simulink model "Han_HQ_Sim_FB"  (Simulink 10.1)
settings: Solver=ode45  StartTime=0.0  StopTime=10  MaxStep=0.1  RelTol=1e-3  EnableMultiTasking=on
InitFcn:
  | AC=23; %Change to your assigned aircraft
  | SC_DynEqns;
  | X0=[U1 tht 0 tht 0 0 0 0]';
  | maneuver = 1;
  | Han_MK_CLAW;
StartFcn:
  | tic
StopFcn:
  | toctime=toc;
  | if maneuver <1.5
  | mkplot_Pitch
  | elseif maneuver <2.5
  | mkplot_Roll
  | else
  | mkplot_Yaw
  | end
undefined symbols (not defined in the file): A, Alt, B, d2r, fps2kt, K, K_pitch, K_roll, K_yaw, P1, P2, P3, pdoub, pdoub_t, r2d, rdoub, rdoub_t, tht, ydoub, ydoub_t, Z1, Z2, Z3
libraries: simulink x42
settings Model: Creator=bordignk  LastModifiedBy=Edward Han
settings DataIOCC: SignalLoggingSaveFormat=ModelDataLogs
settings OptimizationCC: ExpressionDepthLimit=2147483647  InitFltsAndDblsToZero=on
settings DebuggingCC: FcnCallInpInsideContextMsg=warning  UnconnectedInputMsg=none  UnconnectedOutputMsg=none  StateNameClashWarn=warning  SFExecutionAtInitializationDiag=warning
settings SFSimCC: SimParseCustomCode=off
settings ConfigComp: CovSFcnEnable=off

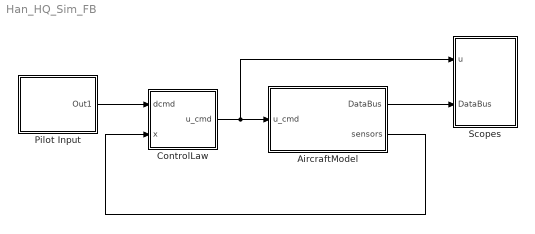
== system Han_HQ_Sim_FB ==
  AircraftModel : Subsystem
  ControlLaw : Subsystem
  Pilot Input : Subsystem
  Scopes : Subsystem
  wires:
  AircraftModel/1(DataBus) -> Scopes/2(DataBus)
  ControlLaw/1(u_cmd) -> AircraftModel/1(u_cmd), Scopes/1(u)
  AircraftModel/2(sensors) -> ControlLaw/2(x)
  Pilot Input/1(Out1) -> ControlLaw/1(dcmd)

== system Han_HQ_Sim_FB/AircraftModel ==
  u_cmd : Inport
  ControlLimits : Subsystem
  Gain : Gain  Gain=B  Multiplication=Matrix(K*u)
  Gain2 : Gain  Gain=A  Multiplication=Matrix(K*u)
  Integrator : Integrator  InitialCondition=zeros(8,1)
  Make_Data : Subsystem
  Sum : Sum  Inputs=|++
  DataBus : Outport
  sensors : Outport  Port=2
  wires:
  Gain2/1 -> Sum/2
  Sum/1 -> Integrator/1, Make_Data/1(xdt)  "xdt"
  Gain/1 -> Sum/1
  u_cmd/1 -> ControlLimits/1(u_cmd)
  Make_Data/1(DataBus) -> DataBus/1
  ControlLimits/1(u) -> Gain/1
  Integrator/1 -> Make_Data/2(x)  "x"
  Make_Data/2(x_out) -> sensors/1, Gain2/1

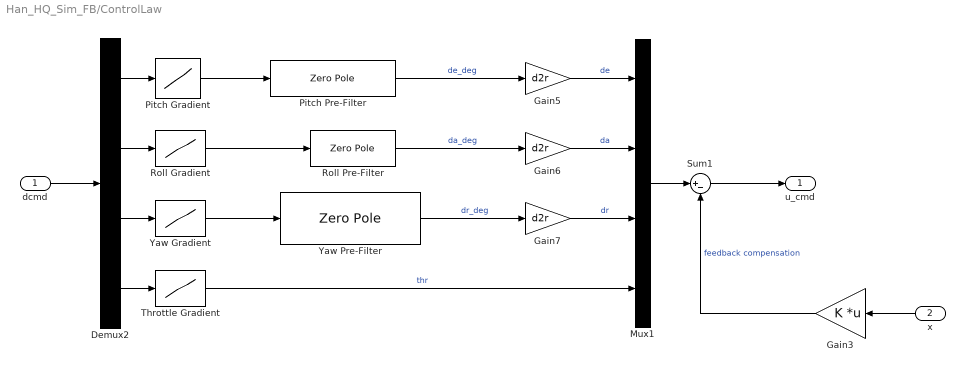
== system Han_HQ_Sim_FB/ControlLaw ==
  dcmd : Inport
  x : Inport  Port=2
  Demux2 : Demux
  Gain3 : Gain  Gain=K  Multiplication=Matrix(K*u)
  Gain5 : Gain  Gain=d2r
  Gain6 : Gain  Gain=d2r
  Gain7 : Gain  Gain=d2r
  Mux1 : Mux
  Pitch Gradient : Lookup  InputValues=[-1 1]  Table=[25 -25]  LookUpMeth=Interpolation-Use End Values
  Pitch Pre-Filter : ZeroPole  Zeros=[P1(3:4)]  Poles=Z1  Gain=K_pitch
  Roll Gradient : Lookup  InputValues=[-1 1]  Table=[-30 30]  LookUpMeth=Interpolation-Use End Values
  Roll Pre-Filter : ZeroPole  Zeros=[P2(4)]  Poles=Z2  Gain=K_roll
  Sum1 : Sum  Inputs=|+-
  Throttle Gradient : Lookup  InputValues=[-1 1]  Table=[5 -5]  LookUpMeth=Interpolation-Use End Values
  Yaw Gradient : Lookup  InputValues=[-1 1]  Table=[-30 30]  LookUpMeth=Interpolation-Use End Values
  Yaw Pre-Filter : ZeroPole  Zeros=[P3(4) P3(3)]  Poles=[Z3]  Gain=K_yaw
  u_cmd : Outport
  wires:
  Gain3/1 -> Sum1/2  "feedback compensation"
  Sum1/1 -> u_cmd/1
  x/1 -> Gain3/1
  Gain6/1 -> Mux1/2  "da"
  Gain7/1 -> Mux1/3  "dr"
  Demux2/2 -> Roll Gradient/1
  Demux2/4 -> Throttle Gradient/1
  Pitch Gradient/1 -> Pitch Pre-Filter/1
  Roll Gradient/1 -> Roll Pre-Filter/1
  Throttle Gradient/1 -> Mux1/4  "thr"
  Gain5/1 -> Mux1/1  "de"
  dcmd/1 -> Demux2/1
  Demux2/1 -> Pitch Gradient/1
  Mux1/1 -> Sum1/1
  Pitch Pre-Filter/1 -> Gain5/1  "de_deg"
  Roll Pre-Filter/1 -> Gain6/1  "da_deg"
  Yaw Gradient/1 -> Yaw Pre-Filter/1
  Demux2/3 -> Yaw Gradient/1
  Yaw Pre-Filter/1 -> Gain7/1  "dr_deg"

== system Han_HQ_Sim_FB/Pilot Input ==
  Mux : Mux
  Pitch Stick Sequence : Subsystem  mask{SEQ_t=pdoub_t, SEQ=pdoub}
      mask prompts: SEQ_t "Time values:"; SEQ "Output values:"
      mask Display: disp('Non-repeating\nSequence')
  Roll Stick Sequence : Subsystem  mask{SEQ_t=rdoub_t, SEQ=rdoub}
      mask prompts: SEQ_t "Time values:"; SEQ "Output values:"
      mask Display: disp('Non-repeating\nSequence')
  Rudder Pedal Sequence : Subsystem  mask{SEQ_t=ydoub_t, SEQ=ydoub}
      mask prompts: SEQ_t "Time values:"; SEQ "Output values:"
      mask Display: disp('Non-repeating\nSequence')
  Throttle Sequence : Subsystem  mask{SEQ_t=[0 25], SEQ=[0 0]}
      mask prompts: SEQ_t "Time values:"; SEQ "Output values:"
      mask Display: disp('Non-repeating\nSequence')
  To Workspace : ToWorkspace  VariableName=pilot_pitch  SampleTime=-1
  To Workspace1 : ToWorkspace  VariableName=pilot_roll  SampleTime=-1
  To Workspace2 : ToWorkspace  VariableName=pilot_rudder  SampleTime=-1
  To Workspace3 : ToWorkspace  VariableName=pilot_throttle  SampleTime=-1
  Out1 : Outport
  wires:
  Mux/1 -> Out1/1
  Pitch Stick Sequence/1(Out1) -> To Workspace/1, Mux/1  "dpitch"
  Rudder Pedal Sequence/1(Out1) -> Mux/3, To Workspace2/1  "dyaw"
  Roll Stick Sequence/1(Out1) -> To Workspace1/1, Mux/2  "droll"
  Throttle Sequence/1(Out1) -> Mux/4, To Workspace3/1  "dthr"

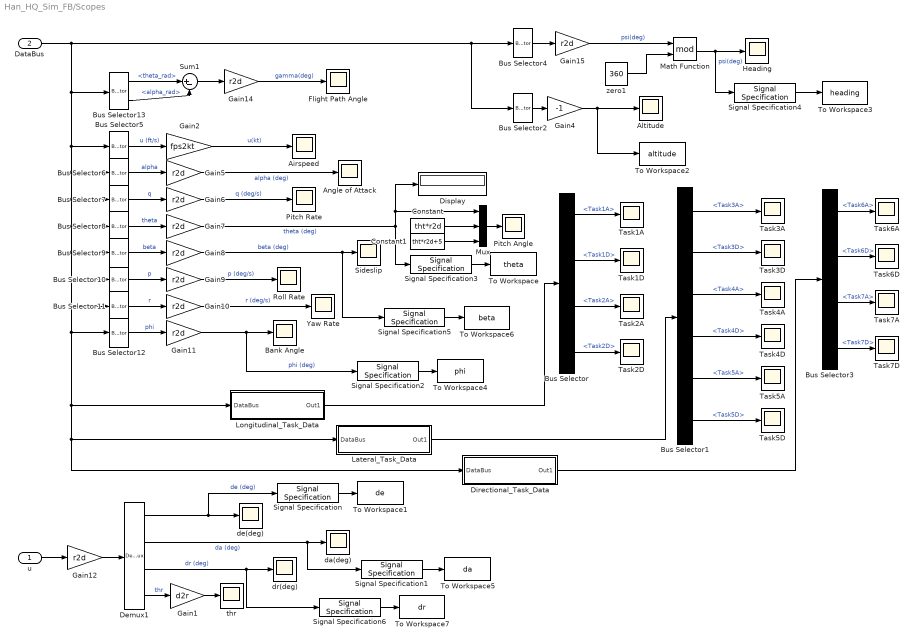
== system Han_HQ_Sim_FB/Scopes ==
  u : Inport
  DataBus : Inport  Port=2
  Airspeed : Scope
  Altitude : Scope
  Angle of Attack : Scope
  Bank Angle : Scope
  Bus Selector : BusSelector  OutputSignals=Task1A,Task1D,Task2A,Task2D
  Bus Selector1 : BusSelector  OutputSignals=Task3A,Task3D,Task4A,Task4D,Task5A,Task5D
  Bus Selector10 : BusSelector  OutputSignals=p_rps  OutputAsBus=on
  Bus Selector11 : BusSelector  OutputSignals=r_rps  OutputAsBus=on
  Bus Selector12 : BusSelector  OutputSignals=phi_rad  OutputAsBus=on
  Bus Selector13 : BusSelector  OutputSignals=theta_rad,alpha_rad
  Bus Selector2 : BusSelector  OutputSignals=ze_ft  OutputAsBus=on
  Bus Selector3 : BusSelector  OutputSignals=Task6A,Task6D,Task7A,Task7D
  Bus Selector4 : BusSelector  OutputSignals=psi_rad  OutputAsBus=on
  Bus Selector5 : BusSelector  OutputSignals=v_fps  OutputAsBus=on
  Bus Selector6 : BusSelector  OutputSignals=alpha_rad  OutputAsBus=on
  Bus Selector7 : BusSelector  OutputSignals=q_rps  OutputAsBus=on
  Bus Selector8 : BusSelector  OutputSignals=theta_rad  OutputAsBus=on
  Bus Selector9 : BusSelector  OutputSignals=beta_rad  OutputAsBus=on
  Constant : Constant  Value=tht*r2d
  Constant1 : Constant  Value=tht*r2d+5
  Demux1 : Demux
  Directional_Task_Data : Subsystem
  Display : Display
  Flight Path Angle : Scope
  Gain1 : Gain  Gain=d2r
  Gain{5..12,14..15} (10 alike) : Gain  Gain=r2d
  Gain2 : Gain  Gain=fps2kt
  Gain4 : Gain  Gain=-1
  Heading : Scope
  Lateral_Task_Data : Subsystem
  Longitudinal_Task_Data : Subsystem
  Math Function : Math  Operator=mod  SignedPower=on  SaturateOnIntegerOverflow=on
  Mux : Mux  Inputs=3
  Pitch Angle : Scope
  Pitch Rate : Scope
  Roll Rate : Scope
  Sideslip : Scope
  Signal Specification{,1..6} (7 alike) : SignalSpecification  Dimensions=[1]
  Sum1 : Sum  Inputs=|+-
  Task1A : Scope
  Task1D : Scope
  Task2A : Scope
  Task2D : Scope
  Task3A : Scope
  Task3D : Scope
  Task4A : Scope
  Task4D : Scope
  Task5A : Scope
  Task5D : Scope
  Task6A : Scope
  Task6D : Scope
  Task7A : Scope
  Task7D : Scope
  To Workspace : ToWorkspace  VariableName=theta  SampleTime=-1
  To Workspace1 : ToWorkspace  VariableName=de  SampleTime=-1
  To Workspace2 : ToWorkspace  VariableName=altitude  SampleTime=-1
  To Workspace3 : ToWorkspace  VariableName=heading  SampleTime=-1
  To Workspace4 : ToWorkspace  VariableName=phi  SampleTime=-1
  To Workspace5 : ToWorkspace  VariableName=da  SampleTime=-1
  To Workspace6 : ToWorkspace  VariableName=beta  SampleTime=-1
  To Workspace7 : ToWorkspace  VariableName=dr  SampleTime=-1
  Yaw Rate : Scope
  da(deg) : Scope
  de(deg) : Scope
  dr(deg) : Scope
  thr : Scope
  zero1 : Constant  Value=360
  wires:
  Gain12/1 -> Demux1/1
  Demux1/1 -> de(deg)/1, Signal Specification/1  "de (deg)"
  Demux1/2 -> da(deg)/1, Signal Specification1/1  "da (deg)"
  Demux1/3 -> dr(deg)/1, Signal Specification6/1  "dr (deg)"
  u/1 -> Gain12/1
  DataBus/1 -> Bus Selector5/1, Bus Selector6/1, Bus Selector7/1, Bus Selector8/1, Bus Selector9/1, Bus Selector10/1, Bus Selector11/1, Bus Selector12/1, Directional_Task_Data/1(DataBus), Lateral_Task_Data/1(DataBus), Longitudinal_Task_Data/1(DataBus), Bus Selector13/1, Bus Selector4/1, Bus Selector2/1
  Demux1/4 -> Gain1/1  "thr"
  Math Function/1 -> Heading/1, Signal Specification4/1  "psi(deg)"
  Bus Selector2/1 -> Gain4/1
  Gain4/1 -> Altitude/1, To Workspace2/1
  Bus Selector4/1 -> Gain15/1
  Bus Selector5/1 -> Gain2/1  "u (ft/s)"
  Bus Selector6/1 -> Gain5/1  "alpha"
  Bus Selector7/1 -> Gain6/1  "q"
  Bus Selector8/1 -> Gain7/1  "theta"
  Bus Selector9/1 -> Gain8/1  "beta"
  Bus Selector10/1 -> Gain9/1  "p"
  Bus Selector11/1 -> Gain10/1  "r"
  Bus Selector12/1 -> Gain11/1  "phi"
  Gain5/1 -> Angle of Attack/1  "alpha (deg)"
  Gain6/1 -> Pitch Rate/1  "q (deg/s)"
  Gain7/1 -> Signal Specification3/1, Display/1, Mux/1  "theta (deg)"
  Gain8/1 -> Sideslip/1, Signal Specification5/1  "beta (deg)"
  Gain9/1 -> Roll Rate/1  "p (deg/s)"
  Gain10/1 -> Yaw Rate/1  "r (deg/s)"
  Gain11/1 -> Bank Angle/1, Signal Specification2/1  "phi (deg)"
  Gain2/1 -> Airspeed/1  "u(kt)"
  Gain1/1 -> thr/1
  Gain15/1 -> Math Function/1  "psi(deg)"
  zero1/1 -> Math Function/2
  Gain14/1 -> Flight Path Angle/1  "gamma(deg)"
  Bus Selector13/1 -> Sum1/1  "<theta_rad>"
  Bus Selector13/2 -> Sum1/2  "<alpha_rad>"
  Sum1/1 -> Gain14/1
  Signal Specification/1 -> To Workspace1/1
  Signal Specification1/1 -> To Workspace5/1
  Signal Specification2/1 -> To Workspace4/1
  Signal Specification3/1 -> To Workspace/1
  Signal Specification4/1 -> To Workspace3/1
  Signal Specification5/1 -> To Workspace6/1
  Signal Specification6/1 -> To Workspace7/1
  Longitudinal_Task_Data/1(Out1) -> Bus Selector/1
  Bus Selector/1 -> Task1A/1  "<Task1A>"
  Bus Selector/2 -> Task1D/1  "<Task1D>"
  Bus Selector/3 -> Task2A/1  "<Task2A>"
  Bus Selector/4 -> Task2D/1  "<Task2D>"
  Lateral_Task_Data/1(Out1) -> Bus Selector1/1
  Bus Selector1/1 -> Task3A/1  "<Task3A>"
  Bus Selector1/2 -> Task3D/1  "<Task3D>"
  Bus Selector1/3 -> Task4A/1  "<Task4A>"
  Bus Selector1/4 -> Task4D/1  "<Task4D>"
  Bus Selector1/5 -> Task5A/1  "<Task5A>"
  Bus Selector1/6 -> Task5D/1  "<Task5D>"
  Directional_Task_Data/1(Out1) -> Bus Selector3/1
  Bus Selector3/1 -> Task6A/1  "<Task6A>"
  Bus Selector3/2 -> Task6D/1  "<Task6D>"
  Bus Selector3/3 -> Task7A/1  "<Task7A>"
  Bus Selector3/4 -> Task7D/1  "<Task7D>"
  Mux/1 -> Pitch Angle/1
  Constant/1 -> Mux/2
  Constant1/1 -> Mux/3

== system Han_HQ_Sim_FB/AircraftModel/ControlLimits ==
  u_cmd : Inport
  Demux2 : Demux
  Mux : Mux
  Saturation : Saturate  UpperLimit=25*d2r  LowerLimit=-25*d2r
  Saturation1 : Saturate  UpperLimit=30*d2r  LowerLimit=-30*d2r
  Saturation2 : Saturate  UpperLimit=30*d2r  LowerLimit=-30*d2r
  Saturation3 : Saturate  UpperLimit=5  LowerLimit=-5
  u : Outport
  wires:
  Demux2/1 -> Saturation/1
  Demux2/2 -> Saturation1/1
  Demux2/3 -> Saturation2/1
  Saturation/1 -> Mux/1
  Saturation1/1 -> Mux/2
  Saturation2/1 -> Mux/3
  Saturation3/1 -> Mux/4
  u_cmd/1 -> Demux2/1
  Mux/1 -> u/1
  Demux2/4 -> Saturation3/1

== system Han_HQ_Sim_FB/AircraftModel/Make_Data ==
  xdt : Inport  PortDimensions=[8 1]
  x : Inport  Port=2  PortDimensions=[8 1]
  Bus Selector : BusSelector  OutputSignals=v_fps,alpha_rad,q_rps,theta_rad,beta_rad,p_rps,r_rps,phi_rad  OutputAsBus=on
  Bus to Vector : BusToVector
  Constant : Constant  Value=X0
  Constant1 : Constant  Value=X0
  Earth Axis : Subsystem
  Subsystem2 : Subsystem
  Sum1 : Sum  Inputs=|++
  Sum2 : Sum  Inputs=|+-
  DataBus : Outport
  x_out : Outport  Port=2
  wires:
  x/1 -> Sum1/1
  Constant/1 -> Sum1/2
  Sum1/1 -> Subsystem2/1(x), Earth Axis/1(x)
  Earth Axis/2(xe) -> Subsystem2/3(Xe)
  xdt/1 -> Subsystem2/4(xdt)
  Subsystem2/1(DataBus) -> Bus Selector/1, DataBus/1
  Earth Axis/1(Ve) -> Subsystem2/2(Ve)
  Bus Selector/1 -> Bus to Vector/1
  Bus to Vector/1 -> Sum2/1
  Constant1/1 -> Sum2/2
  Sum2/1 -> x_out/1

== system Han_HQ_Sim_FB/Pilot Input/Pitch Stick Sequence ==
  Clock : Clock
  Lookup Table : Lookup  InputValues=SEQ_t  Table=SEQ  LookUpMeth=Interpolation-Use End Values
  Out1 : Outport
  wires:
  Clock/1 -> Lookup Table/1
  Lookup Table/1 -> Out1/1

== system Han_HQ_Sim_FB/Pilot Input/Roll Stick Sequence ==
  Clock : Clock
  Lookup Table : Lookup  InputValues=SEQ_t  Table=SEQ  LookUpMeth=Interpolation-Use End Values
  Out1 : Outport
  wires:
  Lookup Table/1 -> Out1/1
  Clock/1 -> Lookup Table/1

== system Han_HQ_Sim_FB/Pilot Input/Rudder Pedal Sequence ==
  Clock : Clock
  Lookup Table : Lookup  InputValues=SEQ_t  Table=SEQ  LookUpMeth=Interpolation-Use End Values
  Out1 : Outport
  wires:
  Clock/1 -> Lookup Table/1
  Lookup Table/1 -> Out1/1

== system Han_HQ_Sim_FB/Pilot Input/Throttle Sequence ==
  Clock : Clock
  Lookup Table : Lookup  InputValues=SEQ_t  Table=SEQ  LookUpMeth=Interpolation-Use End Values
  Out1 : Outport
  wires:
  Lookup Table/1 -> Out1/1
  Clock/1 -> Lookup Table/1

== system Han_HQ_Sim_FB/Scopes/Directional_Task_Data ==
  DataBus : Inport
  Bus Creator : BusCreator  Inputs=4
  Bus Selector1 : BusSelector  OutputSignals=beta_rad
  Gain2 : Gain  Gain=r2d
  Task6 : Subsystem
  Task7 : Subsystem
  Out1 : Outport
  wires:
  Gain2/1 -> Task6/1(In1), Task7/2(In2)  "beta_deg"
  Bus Selector1/1 -> Gain2/1  "<beta_rad>"
  DataBus/1 -> Bus Selector1/1
  Bus Creator/1 -> Out1/1
  Task6/1(Task6D) -> Bus Creator/1
  Task6/2(Task6A) -> Task7/1(In1), Bus Creator/2
  Task7/1(Task7D) -> Bus Creator/3
  Task7/2(Task7A) -> Bus Creator/4

== system Han_HQ_Sim_FB/Scopes/Lateral_Task_Data ==
  DataBus : Inport
  Bus Creator : BusCreator  Inputs=6
  Bus Selector1 : BusSelector  OutputSignals=phi_rad
  Gain2 : Gain  Gain=r2d
  Task3 : Subsystem
  Task4 : Subsystem
  Task5 : Subsystem
  Out1 : Outport
  wires:
  DataBus/1 -> Bus Selector1/1
  Bus Selector1/1 -> Gain2/1  "<phi_rad>"
  Gain2/1 -> Task3/1(In1), Task4/2(In2), Task5/2(In2)  "phi_deg"
  Task3/2(Task3A) -> Task4/1(In1), Bus Creator/2
  Bus Creator/1 -> Out1/1
  Task3/1(Task3D) -> Bus Creator/1
  Task4/1(Task4D) -> Bus Creator/3
  Task5/1(Task5A) -> Bus Creator/5
  Task5/2(Task5D) -> Bus Creator/6
  Task4/2(Task4A) -> Task5/1(In1), Bus Creator/4

== system Han_HQ_Sim_FB/Scopes/Longitudinal_Task_Data ==
  DataBus : Inport
  Bus Creator : BusCreator  Inputs=4
  Bus Selector1 : BusSelector  OutputSignals=theta_rad  OutputAsBus=on
  Gain6 : Gain  Gain=r2d
  Task1 : Subsystem
  Task2 : Subsystem
  Out1 : Outport
  wires:
  DataBus/1 -> Bus Selector1/1
  Bus Selector1/1 -> Gain6/1
  Gain6/1 -> Task1/1(In1), Task2/2(In1)
  Task1/2(Task1A) -> Task2/1(In2), Bus Creator/2
  Task2/1(Task2A) -> Bus Creator/3
  Task2/2(Task2D) -> Bus Creator/4
  Bus Creator/1 -> Out1/1
  Task1/1(Task1D) -> Bus Creator/1

== system Han_HQ_Sim_FB/AircraftModel/Make_Data/Earth Axis ==
  x : Inport
  Selector : Selector  InputPortWidth=8  IndexOptions=Index vector (dialog)  Indices=[6 3 7]  OutputSizes=1
  Subsystem : Subsystem
  Subsystem1 : Subsystem
  Transpose : Math  Operator=transpose  SignedPower=on  SaturateOnIntegerOverflow=on
  uvw_body : Subsystem
  xe,ye,ze : Integrator  InitialCondition=[0 0 -Alt]
  Ve : Outport
  xe : Outport  Port=2
  wires:
  Subsystem1/1(DCM) -> Transpose/1
  Transpose/1 -> Subsystem/2(transform coefficients)
  Selector/1 -> Subsystem1/1("p q r ")
  uvw_body/1(Out1) -> Subsystem/1(x y z)
  x/1 -> Selector/1, uvw_body/1(In1)
  xe,ye,ze/1 -> xe/1
  Subsystem/1(Ve1) -> Ve/1, xe,ye,ze/1

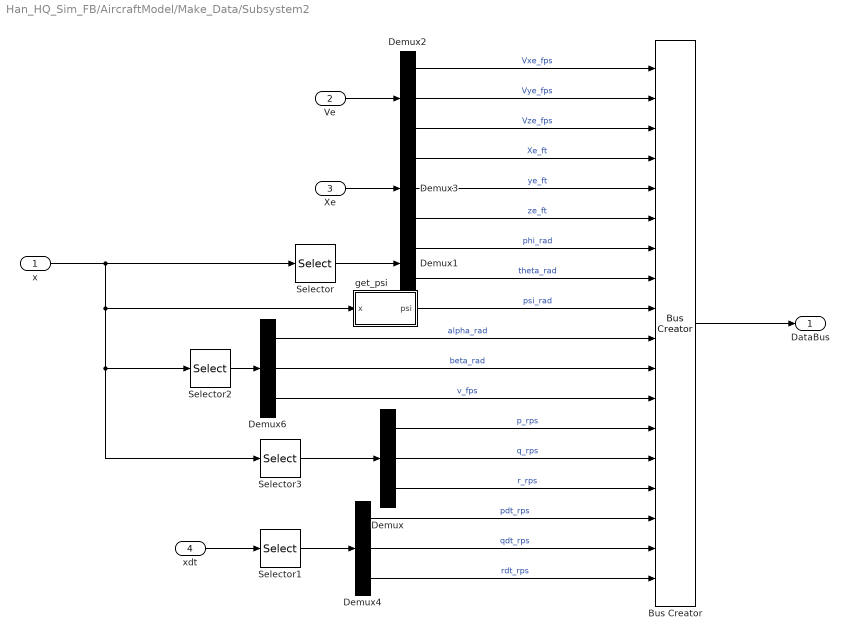
== system Han_HQ_Sim_FB/AircraftModel/Make_Data/Subsystem2 ==
  x : Inport
  Ve : Inport  Port=2
  Xe : Inport  Port=3
  xdt : Inport  Port=4
  Bus Creator : BusCreator  Inputs=18
  Demux{,2..4,6} (5 alike) : Demux  Outputs=3
  Demux1 : Demux  Outputs=2
  Selector : Selector  InputPortWidth=8  IndexOptions=Index vector (dialog)  Indices=[8 4]  OutputSizes=1
  Selector1 : Selector  InputPortWidth=8  IndexOptions=Index vector (dialog)  Indices=[6 3 7]  OutputSizes=1
  Selector2 : Selector  InputPortWidth=8  IndexOptions=Index vector (dialog)  Indices=[2 5 1]  OutputSizes=1
  Selector3 : Selector  InputPortWidth=8  IndexOptions=Index vector (dialog)  Indices=[6 3 7]  OutputSizes=1
  get_psi : Subsystem
  DataBus : Outport
  wires:
  Selector2/1 -> Demux6/1
  Selector/1 -> Demux1/1
  x/1 -> get_psi/1(x), Selector3/1, Selector2/1, Selector/1
  Demux4/3 -> Bus Creator/18  "rdt_rps"
  Demux4/2 -> Bus Creator/17  "qdt_rps"
  Demux4/1 -> Bus Creator/16  "pdt_rps"
  Demux/3 -> Bus Creator/15  "r_rps"
  Demux/2 -> Bus Creator/14  "q_rps"
  Demux/1 -> Bus Creator/13  "p_rps"
  Demux6/3 -> Bus Creator/12  "v_fps"
  Demux6/2 -> Bus Creator/11  "beta_rad"
  Demux6/1 -> Bus Creator/10  "alpha_rad"
  get_psi/1(psi) -> Bus Creator/9  "psi_rad"
  Demux1/2 -> Bus Creator/8  "theta_rad"
  Demux1/1 -> Bus Creator/7  "phi_rad"
  Demux3/3 -> Bus Creator/6  "ze_ft"
  Demux3/2 -> Bus Creator/5  "ye_ft"
  Demux3/1 -> Bus Creator/4  "Xe_ft"
  Demux2/3 -> Bus Creator/3  "Vze_fps"
  Demux2/2 -> Bus Creator/2  "Vye_fps"
  Demux2/1 -> Bus Creator/1  "Vxe_fps"
  xdt/1 -> Selector1/1
  Xe/1 -> Demux3/1
  Ve/1 -> Demux2/1
  Bus Creator/1 -> DataBus/1
  Selector3/1 -> Demux/1
  Selector1/1 -> Demux4/1

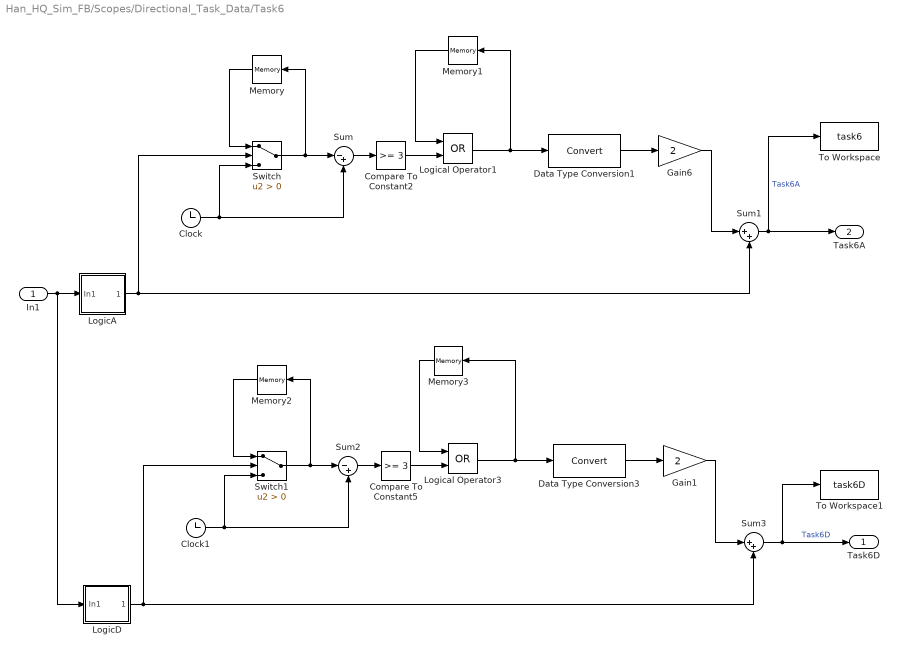
== system Han_HQ_Sim_FB/Scopes/Directional_Task_Data/Task6 ==
  In1 : Inport
  Clock : Clock
  Clock1 : Clock
  Compare To Constant2 : simulink/Logic and Bit Operations/Compare To Constant  relop=>=  const=3  OutDataTypeStr=uint8  ZeroCross=off
  Compare To Constant5 : simulink/Logic and Bit Operations/Compare To Constant  relop=>=  const=3  OutDataTypeStr=uint8  ZeroCross=off
  Data Type Conversion1 : DataTypeConversion
  Data Type Conversion3 : DataTypeConversion
  Gain1 : Gain  Gain=2
  Gain6 : Gain  Gain=2
  LogicA : Subsystem
  LogicD : Subsystem
  Logical Operator1 : Logic  Operator=OR  AllPortsSameDT=off  OutDataTypeStr=boolean
  Logical Operator3 : Logic  Operator=OR  AllPortsSameDT=off  OutDataTypeStr=boolean
  Memory{,1..3} (4 alike) : Memory
  Sum : Sum  Inputs=|-+
  Sum1 : Sum  Inputs=|++
  Sum2 : Sum  Inputs=|-+
  Sum3 : Sum  Inputs=|++
  Switch : Switch  Criteria=u2 > Threshold
  Switch1 : Switch  Criteria=u2 > Threshold
  To Workspace : ToWorkspace  VariableName=task6  SampleTime=-1
  To Workspace1 : ToWorkspace  VariableName=task6D  SampleTime=-1
  Task6D : Outport
  Task6A : Outport  Port=2
  wires:
  LogicD/1(Out1) -> Switch1/2, Sum3/2
  Gain1/1 -> Sum3/1
  Data Type Conversion3/1 -> Gain1/1
  Sum3/1 -> To Workspace1/1, Task6D/1  "Task6D"
  Memory3/1 -> Logical Operator3/1
  Logical Operator3/1 -> Memory3/1, Data Type Conversion3/1
  Compare To Constant5/1 -> Logical Operator3/2
  Sum2/1 -> Compare To Constant5/1
  Memory2/1 -> Switch1/1
  Switch1/1 -> Sum2/1, Memory2/1
  Clock1/1 -> Sum2/2, Switch1/3
  LogicA/1(Out1) -> Switch/2, Sum1/2
  Gain6/1 -> Sum1/1
  Data Type Conversion1/1 -> Gain6/1
  Sum1/1 -> Task6A/1, To Workspace/1  "Task6A"
  Memory1/1 -> Logical Operator1/1
  Logical Operator1/1 -> Memory1/1, Data Type Conversion1/1
  Compare To Constant2/1 -> Logical Operator1/2
  Sum/1 -> Compare To Constant2/1
  Memory/1 -> Switch/1
  Switch/1 -> Sum/1, Memory/1
  Clock/1 -> Sum/2, Switch/3
  In1/1 -> LogicD/1(In1), LogicA/1(In1)

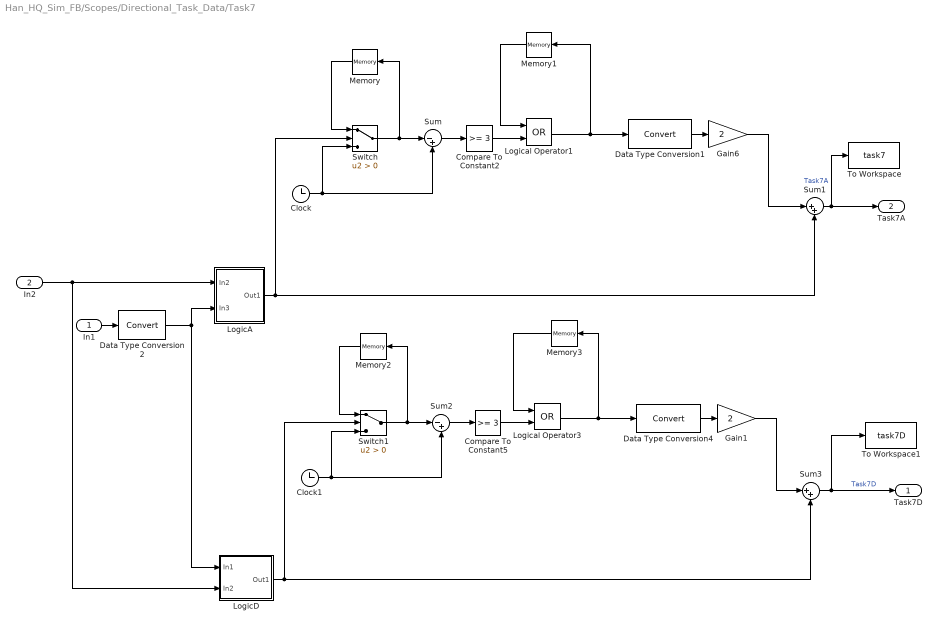
== system Han_HQ_Sim_FB/Scopes/Directional_Task_Data/Task7 ==
  In1 : Inport
  In2 : Inport  Port=2
  Clock : Clock
  Clock1 : Clock
  Compare To Constant2 : simulink/Logic and Bit Operations/Compare To Constant  relop=>=  const=3  OutDataTypeStr=uint8  ZeroCross=off
  Compare To Constant5 : simulink/Logic and Bit Operations/Compare To Constant  relop=>=  const=3  OutDataTypeStr=uint8  ZeroCross=off
  Data Type Conversion1 : DataTypeConversion
  Data Type Conversion2 : DataTypeConversion
  Data Type Conversion4 : DataTypeConversion
  Gain1 : Gain  Gain=2
  Gain6 : Gain  Gain=2
  LogicA : Subsystem
  LogicD : Subsystem
  Logical Operator1 : Logic  Operator=OR  AllPortsSameDT=off  OutDataTypeStr=boolean
  Logical Operator3 : Logic  Operator=OR  AllPortsSameDT=off  OutDataTypeStr=boolean
  Memory{,1..3} (4 alike) : Memory
  Sum : Sum  Inputs=|-+
  Sum1 : Sum  Inputs=|++
  Sum2 : Sum  Inputs=|-+
  Sum3 : Sum  Inputs=|++
  Switch : Switch  Criteria=u2 > Threshold
  Switch1 : Switch  Criteria=u2 > Threshold
  To Workspace : ToWorkspace  VariableName=task7  SampleTime=-1
  To Workspace1 : ToWorkspace  VariableName=task7D  SampleTime=-1
  Task7D : Outport
  Task7A : Outport  Port=2
  wires:
  Gain1/1 -> Sum3/1
  Data Type Conversion4/1 -> Gain1/1
  Sum3/1 -> To Workspace1/1, Task7D/1  "Task7D"
  Memory3/1 -> Logical Operator3/1
  Logical Operator3/1 -> Memory3/1, Data Type Conversion4/1
  Compare To Constant5/1 -> Logical Operator3/2
  Sum2/1 -> Compare To Constant5/1
  Memory2/1 -> Switch1/1
  Switch1/1 -> Sum2/1, Memory2/1
  Clock1/1 -> Sum2/2, Switch1/3
  LogicD/1(Out1) -> Sum3/2, Switch1/2
  Data Type Conversion2/1 -> LogicA/2(In3), LogicD/1(In1)
  Gain6/1 -> Sum1/1
  Data Type Conversion1/1 -> Gain6/1
  In1/1 -> Data Type Conversion2/1
  Sum1/1 -> To Workspace/1, Task7A/1  "Task7A"
  Memory1/1 -> Logical Operator1/1
  Logical Operator1/1 -> Memory1/1, Data Type Conversion1/1
  Compare To Constant2/1 -> Logical Operator1/2
  Sum/1 -> Compare To Constant2/1
  Memory/1 -> Switch/1
  Switch/1 -> Sum/1, Memory/1
  Clock/1 -> Sum/2, Switch/3
  In2/1 -> LogicD/2(In2), LogicA/1(In2)
  LogicA/1(Out1) -> Sum1/2, Switch/2

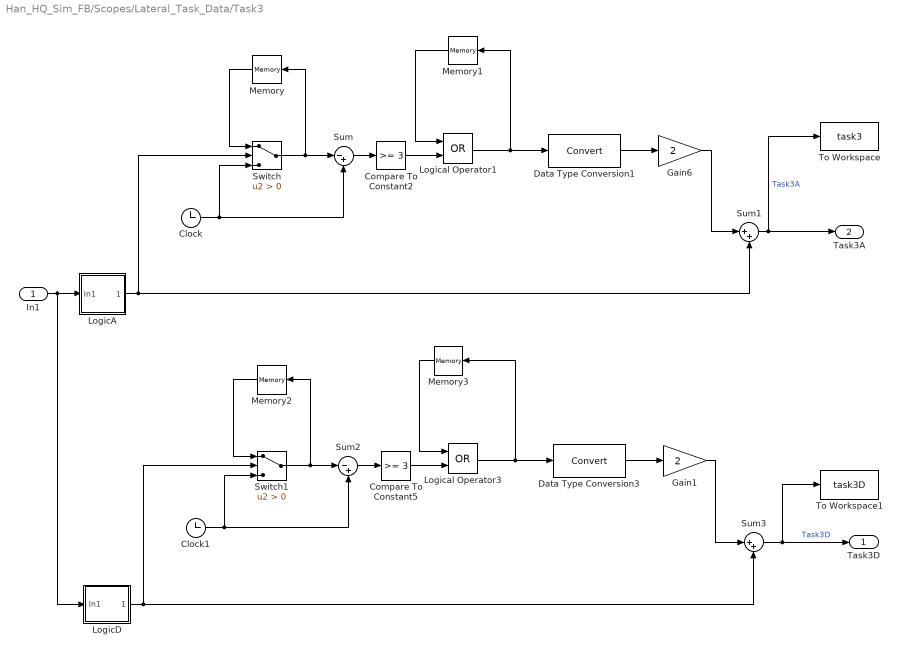
== system Han_HQ_Sim_FB/Scopes/Lateral_Task_Data/Task3 ==
  In1 : Inport
  Clock : Clock
  Clock1 : Clock
  Compare To Constant2 : simulink/Logic and Bit Operations/Compare To Constant  relop=>=  const=3  OutDataTypeStr=uint8  ZeroCross=off
  Compare To Constant5 : simulink/Logic and Bit Operations/Compare To Constant  relop=>=  const=3  OutDataTypeStr=uint8  ZeroCross=off
  Data Type Conversion1 : DataTypeConversion
  Data Type Conversion3 : DataTypeConversion
  Gain1 : Gain  Gain=2
  Gain6 : Gain  Gain=2
  LogicA : Subsystem
  LogicD : Subsystem
  Logical Operator1 : Logic  Operator=OR  AllPortsSameDT=off  OutDataTypeStr=boolean
  Logical Operator3 : Logic  Operator=OR  AllPortsSameDT=off  OutDataTypeStr=boolean
  Memory{,1..3} (4 alike) : Memory
  Sum : Sum  Inputs=|-+
  Sum1 : Sum  Inputs=|++
  Sum2 : Sum  Inputs=|-+
  Sum3 : Sum  Inputs=|++
  Switch : Switch  Criteria=u2 > Threshold
  Switch1 : Switch  Criteria=u2 > Threshold
  To Workspace : ToWorkspace  VariableName=task3  SampleTime=-1
  To Workspace1 : ToWorkspace  VariableName=task3D  SampleTime=-1
  Task3D : Outport
  Task3A : Outport  Port=2
  wires:
  In1/1 -> LogicA/1(In1), LogicD/1(In1)
  Clock/1 -> Switch/3, Sum/2
  Switch/1 -> Memory/1, Sum/1
  Memory/1 -> Switch/1
  Sum/1 -> Compare To Constant2/1
  Compare To Constant2/1 -> Logical Operator1/2
  Logical Operator1/1 -> Data Type Conversion1/1, Memory1/1
  Memory1/1 -> Logical Operator1/1
  Sum1/1 -> Task3A/1, To Workspace/1  "Task3A"
  Data Type Conversion1/1 -> Gain6/1
  Gain6/1 -> Sum1/1
  LogicA/1(Out1) -> Sum1/2, Switch/2
  Clock1/1 -> Switch1/3, Sum2/2
  Switch1/1 -> Memory2/1, Sum2/1
  Memory2/1 -> Switch1/1
  Sum2/1 -> Compare To Constant5/1
  Compare To Constant5/1 -> Logical Operator3/2
  Logical Operator3/1 -> Data Type Conversion3/1, Memory3/1
  Memory3/1 -> Logical Operator3/1
  Sum3/1 -> To Workspace1/1, Task3D/1  "Task3D"
  Data Type Conversion3/1 -> Gain1/1
  Gain1/1 -> Sum3/1
  LogicD/1(Out1) -> Sum3/2, Switch1/2

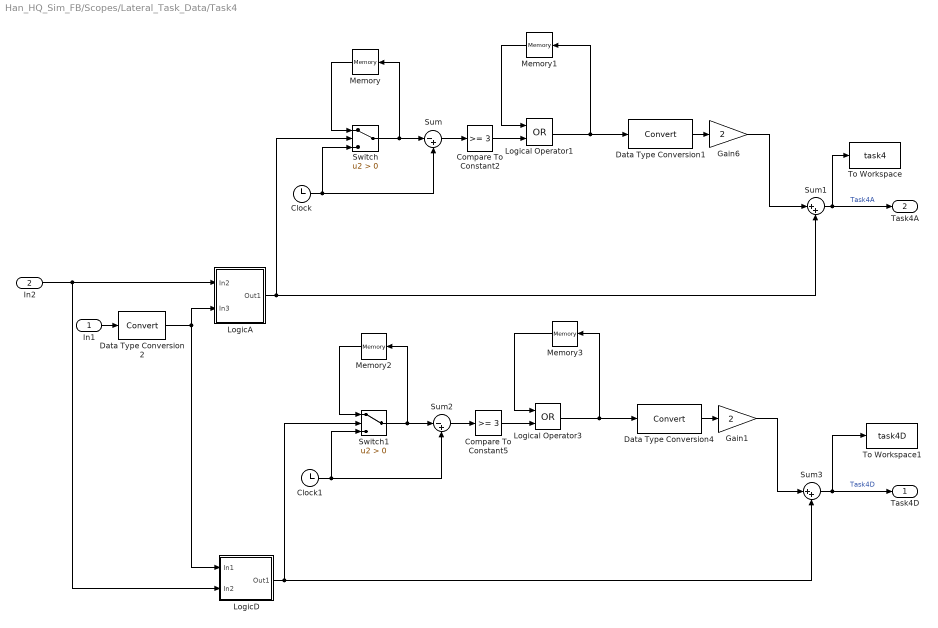
== system Han_HQ_Sim_FB/Scopes/Lateral_Task_Data/Task4 ==
  In1 : Inport
  In2 : Inport  Port=2
  Clock : Clock
  Clock1 : Clock
  Compare To Constant2 : simulink/Logic and Bit Operations/Compare To Constant  relop=>=  const=3  OutDataTypeStr=uint8  ZeroCross=off
  Compare To Constant5 : simulink/Logic and Bit Operations/Compare To Constant  relop=>=  const=3  OutDataTypeStr=uint8  ZeroCross=off
  Data Type Conversion1 : DataTypeConversion
  Data Type Conversion2 : DataTypeConversion
  Data Type Conversion4 : DataTypeConversion
  Gain1 : Gain  Gain=2
  Gain6 : Gain  Gain=2
  LogicA : Subsystem
  LogicD : Subsystem
  Logical Operator1 : Logic  Operator=OR  AllPortsSameDT=off  OutDataTypeStr=boolean
  Logical Operator3 : Logic  Operator=OR  AllPortsSameDT=off  OutDataTypeStr=boolean
  Memory{,1..3} (4 alike) : Memory
  Sum : Sum  Inputs=|-+
  Sum1 : Sum  Inputs=|++
  Sum2 : Sum  Inputs=|-+
  Sum3 : Sum  Inputs=|++
  Switch : Switch  Criteria=u2 > Threshold
  Switch1 : Switch  Criteria=u2 > Threshold
  To Workspace : ToWorkspace  VariableName=task4  SampleTime=-1
  To Workspace1 : ToWorkspace  VariableName=task4D  SampleTime=-1
  Task4D : Outport
  Task4A : Outport  Port=2
  wires:
  LogicA/1(Out1) -> Switch/2, Sum1/2
  In2/1 -> LogicA/1(In2), LogicD/2(In2)
  Clock/1 -> Switch/3, Sum/2
  Switch/1 -> Memory/1, Sum/1
  Memory/1 -> Switch/1
  Sum/1 -> Compare To Constant2/1
  Compare To Constant2/1 -> Logical Operator1/2
  Logical Operator1/1 -> Data Type Conversion1/1, Memory1/1
  Memory1/1 -> Logical Operator1/1
  Sum1/1 -> To Workspace/1, Task4A/1  "Task4A"
  In1/1 -> Data Type Conversion2/1
  Data Type Conversion1/1 -> Gain6/1
  Gain6/1 -> Sum1/1
  Data Type Conversion2/1 -> LogicD/1(In1), LogicA/2(In3)
  LogicD/1(Out1) -> Switch1/2, Sum3/2
  Clock1/1 -> Switch1/3, Sum2/2
  Switch1/1 -> Memory2/1, Sum2/1
  Memory2/1 -> Switch1/1
  Sum2/1 -> Compare To Constant5/1
  Compare To Constant5/1 -> Logical Operator3/2
  Logical Operator3/1 -> Data Type Conversion4/1, Memory3/1
  Memory3/1 -> Logical Operator3/1
  Sum3/1 -> To Workspace1/1, Task4D/1  "Task4D"
  Data Type Conversion4/1 -> Gain1/1
  Gain1/1 -> Sum3/1

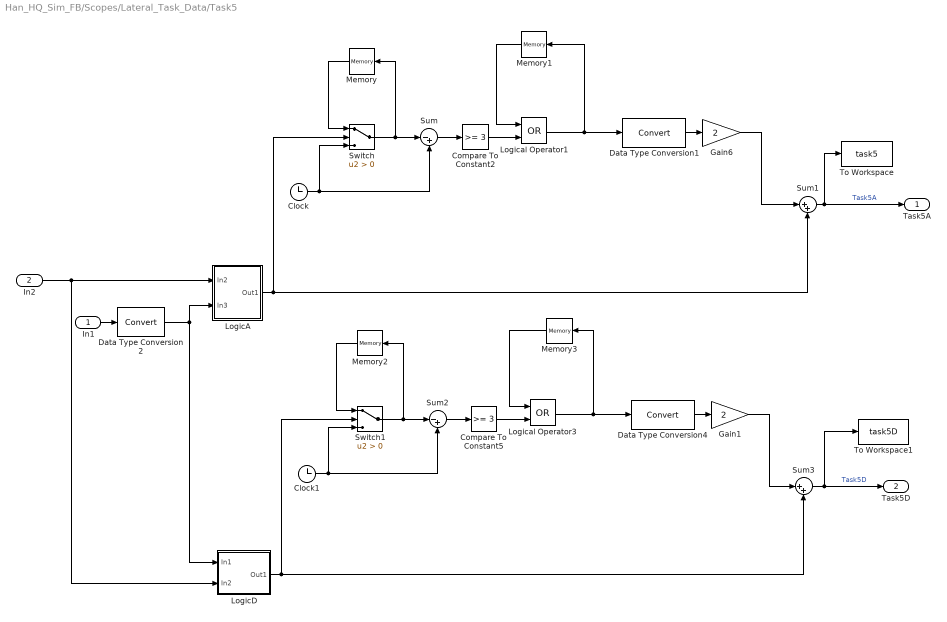
== system Han_HQ_Sim_FB/Scopes/Lateral_Task_Data/Task5 ==
  In1 : Inport
  In2 : Inport  Port=2
  Clock : Clock
  Clock1 : Clock
  Compare To Constant2 : simulink/Logic and Bit Operations/Compare To Constant  relop=>=  const=3  OutDataTypeStr=uint8  ZeroCross=off
  Compare To Constant5 : simulink/Logic and Bit Operations/Compare To Constant  relop=>=  const=3  OutDataTypeStr=uint8  ZeroCross=off
  Data Type Conversion1 : DataTypeConversion
  Data Type Conversion2 : DataTypeConversion
  Data Type Conversion4 : DataTypeConversion
  Gain1 : Gain  Gain=2
  Gain6 : Gain  Gain=2
  LogicA : Subsystem
  LogicD : Subsystem
  Logical Operator1 : Logic  Operator=OR  AllPortsSameDT=off  OutDataTypeStr=boolean
  Logical Operator3 : Logic  Operator=OR  AllPortsSameDT=off  OutDataTypeStr=boolean
  Memory{,1..3} (4 alike) : Memory
  Sum : Sum  Inputs=|-+
  Sum1 : Sum  Inputs=|++
  Sum2 : Sum  Inputs=|-+
  Sum3 : Sum  Inputs=|++
  Switch : Switch  Criteria=u2 > Threshold
  Switch1 : Switch  Criteria=u2 > Threshold
  To Workspace : ToWorkspace  VariableName=task5  SampleTime=-1
  To Workspace1 : ToWorkspace  VariableName=task5D  SampleTime=-1
  Task5A : Outport
  Task5D : Outport  Port=2
  wires:
  LogicA/1(Out1) -> Switch/2, Sum1/2
  In2/1 -> LogicA/1(In2), LogicD/2(In2)
  Clock/1 -> Switch/3, Sum/2
  Switch/1 -> Memory/1, Sum/1
  Memory/1 -> Switch/1
  Sum/1 -> Compare To Constant2/1
  Compare To Constant2/1 -> Logical Operator1/2
  Logical Operator1/1 -> Data Type Conversion1/1, Memory1/1
  Memory1/1 -> Logical Operator1/1
  Sum1/1 -> To Workspace/1, Task5A/1  "Task5A"
  In1/1 -> Data Type Conversion2/1
  Data Type Conversion1/1 -> Gain6/1
  Gain6/1 -> Sum1/1
  Data Type Conversion2/1 -> LogicD/1(In1), LogicA/2(In3)
  LogicD/1(Out1) -> Switch1/2, Sum3/2
  Clock1/1 -> Switch1/3, Sum2/2
  Switch1/1 -> Memory2/1, Sum2/1
  Memory2/1 -> Switch1/1
  Sum2/1 -> Compare To Constant5/1
  Compare To Constant5/1 -> Logical Operator3/2
  Logical Operator3/1 -> Data Type Conversion4/1, Memory3/1
  Memory3/1 -> Logical Operator3/1
  Sum3/1 -> To Workspace1/1, Task5D/1  "Task5D"
  Data Type Conversion4/1 -> Gain1/1
  Gain1/1 -> Sum3/1

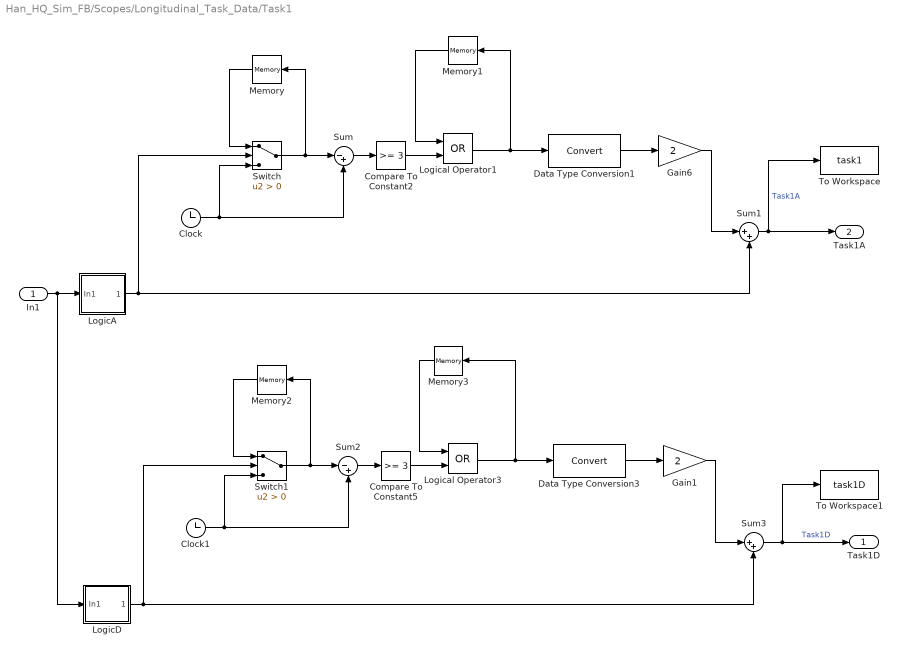
== system Han_HQ_Sim_FB/Scopes/Longitudinal_Task_Data/Task1 ==
  In1 : Inport
  Clock : Clock
  Clock1 : Clock
  Compare To Constant2 : simulink/Logic and Bit Operations/Compare To Constant  relop=>=  const=3  OutDataTypeStr=uint8  ZeroCross=off
  Compare To Constant5 : simulink/Logic and Bit Operations/Compare To Constant  relop=>=  const=3  OutDataTypeStr=uint8  ZeroCross=off
  Data Type Conversion1 : DataTypeConversion
  Data Type Conversion3 : DataTypeConversion
  Gain1 : Gain  Gain=2
  Gain6 : Gain  Gain=2
  LogicA : Subsystem
  LogicD : Subsystem
  Logical Operator1 : Logic  Operator=OR  AllPortsSameDT=off  OutDataTypeStr=boolean
  Logical Operator3 : Logic  Operator=OR  AllPortsSameDT=off  OutDataTypeStr=boolean
  Memory{,1..3} (4 alike) : Memory
  Sum : Sum  Inputs=|-+
  Sum1 : Sum  Inputs=|++
  Sum2 : Sum  Inputs=|-+
  Sum3 : Sum  Inputs=|++
  Switch : Switch  Criteria=u2 > Threshold
  Switch1 : Switch  Criteria=u2 > Threshold
  To Workspace : ToWorkspace  VariableName=task1  SampleTime=-1
  To Workspace1 : ToWorkspace  VariableName=task1D  SampleTime=-1
  Task1D : Outport
  Task1A : Outport  Port=2
  wires:
  In1/1 -> LogicA/1(In1), LogicD/1(In1)
  Clock/1 -> Switch/3, Sum/2
  Switch/1 -> Memory/1, Sum/1
  Memory/1 -> Switch/1
  Sum/1 -> Compare To Constant2/1
  Compare To Constant2/1 -> Logical Operator1/2
  Logical Operator1/1 -> Data Type Conversion1/1, Memory1/1
  Memory1/1 -> Logical Operator1/1
  Sum1/1 -> Task1A/1, To Workspace/1  "Task1A"
  Data Type Conversion1/1 -> Gain6/1
  Gain6/1 -> Sum1/1
  LogicA/1(Out1) -> Sum1/2, Switch/2
  Clock1/1 -> Switch1/3, Sum2/2
  Switch1/1 -> Memory2/1, Sum2/1
  Memory2/1 -> Switch1/1
  Sum2/1 -> Compare To Constant5/1
  Compare To Constant5/1 -> Logical Operator3/2
  Logical Operator3/1 -> Data Type Conversion3/1, Memory3/1
  Memory3/1 -> Logical Operator3/1
  Sum3/1 -> To Workspace1/1, Task1D/1  "Task1D"
  Data Type Conversion3/1 -> Gain1/1
  Gain1/1 -> Sum3/1
  LogicD/1(Out1) -> Sum3/2, Switch1/2

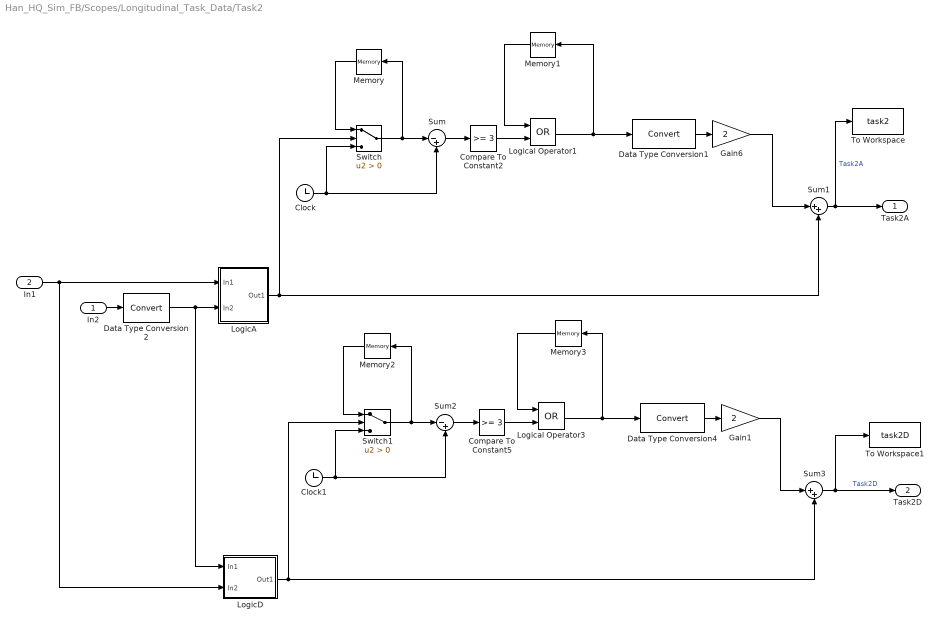
== system Han_HQ_Sim_FB/Scopes/Longitudinal_Task_Data/Task2 ==
  In2 : Inport
  In1 : Inport  Port=2
  Clock : Clock
  Clock1 : Clock
  Compare To Constant2 : simulink/Logic and Bit Operations/Compare To Constant  relop=>=  const=3  OutDataTypeStr=uint8  ZeroCross=off
  Compare To Constant5 : simulink/Logic and Bit Operations/Compare To Constant  relop=>=  const=3  OutDataTypeStr=uint8  ZeroCross=off
  Data Type Conversion1 : DataTypeConversion
  Data Type Conversion2 : DataTypeConversion
  Data Type Conversion4 : DataTypeConversion
  Gain1 : Gain  Gain=2
  Gain6 : Gain  Gain=2
  LogicA : Subsystem
  LogicD : Subsystem
  Logical Operator1 : Logic  Operator=OR  AllPortsSameDT=off  OutDataTypeStr=boolean
  Logical Operator3 : Logic  Operator=OR  AllPortsSameDT=off  OutDataTypeStr=boolean
  Memory{,1..3} (4 alike) : Memory
  Sum : Sum  Inputs=|-+
  Sum1 : Sum  Inputs=|++
  Sum2 : Sum  Inputs=|-+
  Sum3 : Sum  Inputs=|++
  Switch : Switch  Criteria=u2 > Threshold
  Switch1 : Switch  Criteria=u2 > Threshold
  To Workspace : ToWorkspace  VariableName=task2  SampleTime=-1
  To Workspace1 : ToWorkspace  VariableName=task2D  SampleTime=-1
  Task2A : Outport
  Task2D : Outport  Port=2
  wires:
  LogicA/1(Out1) -> Switch/2, Sum1/2
  In1/1 -> LogicA/1(In1), LogicD/2(In2)
  Clock/1 -> Switch/3, Sum/2
  Switch/1 -> Memory/1, Sum/1
  Memory/1 -> Switch/1
  Sum/1 -> Compare To Constant2/1
  Compare To Constant2/1 -> Logical Operator1/2
  Logical Operator1/1 -> Data Type Conversion1/1, Memory1/1
  Memory1/1 -> Logical Operator1/1
  Sum1/1 -> Task2A/1, To Workspace/1  "Task2A"
  In2/1 -> Data Type Conversion2/1
  Data Type Conversion1/1 -> Gain6/1
  Gain6/1 -> Sum1/1
  Data Type Conversion2/1 -> LogicA/2(In2), LogicD/1(In1)
  LogicD/1(Out1) -> Switch1/2, Sum3/2
  Clock1/1 -> Switch1/3, Sum2/2
  Switch1/1 -> Memory2/1, Sum2/1
  Memory2/1 -> Switch1/1
  Sum2/1 -> Compare To Constant5/1
  Compare To Constant5/1 -> Logical Operator3/2
  Logical Operator3/1 -> Data Type Conversion4/1, Memory3/1
  Memory3/1 -> Logical Operator3/1
  Sum3/1 -> Task2D/1, To Workspace1/1  "Task2D"
  Data Type Conversion4/1 -> Gain1/1
  Gain1/1 -> Sum3/1

== system Han_HQ_Sim_FB/AircraftModel/Make_Data/Earth Axis/Subsystem ==
  x y z : Inport
  transform coefficients : Inport  Port=2
  Product : Product  Multiplication=Matrix(*)  InputSameDT=on  SaturateOnIntegerOverflow=on  OutDataTypeStr=Inherit: Same as first input
  Reshape1 : Reshape  OutputDimensionality=Column vector (2-D)
  Reshape2 : Reshape
  Ve1 : Outport
  wires:
  Reshape2/1 -> Ve1/1
  Reshape1/1 -> Product/2
  x y z/1 -> Reshape1/1
  transform coefficients/1 -> Product/1
  Product/1 -> Reshape2/1

== system Han_HQ_Sim_FB/AircraftModel/Make_Data/Earth Axis/Subsystem1 ==
  "p q r " : Inport
  Euler Rates : Subsystem
  Make DCM : Subsystem
  Selector1 : Selector  InputPortWidth=3  IndexOptions=Index vector (dialog)  Indices=[3 2 1]  OutputSizes=1
  phi theta psi : Integrator  InitialCondition=[0 tht pi/2]
  DCM : Outport
  wires:
  Selector1/1 -> Make DCM/1(In1)
  phi theta psi/1 -> Selector1/1, Euler Rates/2(phi theta psi1)
  Euler Rates/1(phidot thetadot psi) -> phi theta psi/1
  "p q r "/1 -> Euler Rates/1(p q r)
  Make DCM/1(Out1) -> DCM/1

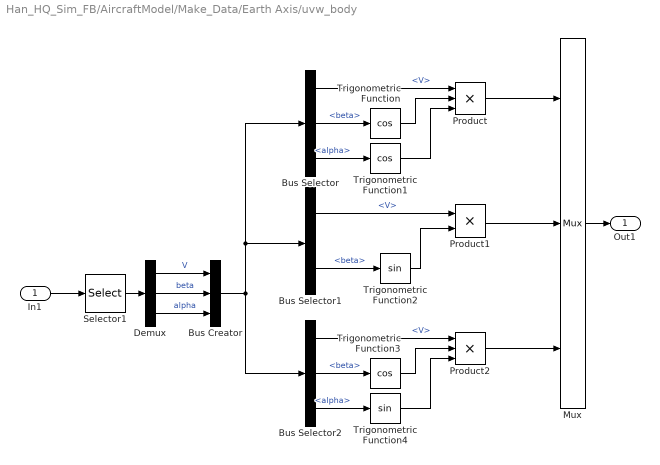
== system Han_HQ_Sim_FB/AircraftModel/Make_Data/Earth Axis/uvw_body ==
  In1 : Inport
  Bus Creator : BusCreator  Inputs=3
  Bus Selector : BusSelector  OutputSignals=V,beta,alpha
  Bus Selector1 : BusSelector  OutputSignals=V,beta
  Bus Selector2 : BusSelector  OutputSignals=V,beta,alpha
  Demux : Demux  Outputs=3
  Mux : Mux  Inputs=3
  Product : Product  Inputs=3  RndMeth=Zero
  Product1 : Product  RndMeth=Zero
  Product2 : Product  Inputs=3  RndMeth=Zero
  Selector1 : Selector  InputPortWidth=8  IndexOptions=Index vector (dialog)  Indices=[1 5 2]  OutputSizes=1
  Trigonometric Function : Trigonometry  Operator=cos
  Trigonometric Function1 : Trigonometry  Operator=cos
  Trigonometric Function2 : Trigonometry
  Trigonometric Function3 : Trigonometry  Operator=cos
  Trigonometric Function4 : Trigonometry
  Out1 : Outport
  wires:
  Selector1/1 -> Demux/1
  Demux/1 -> Bus Creator/1  "V"
  Demux/2 -> Bus Creator/2  "beta"
  Demux/3 -> Bus Creator/3  "alpha"
  Bus Creator/1 -> Bus Selector/1, Bus Selector1/1, Bus Selector2/1
  Bus Selector/2 -> Trigonometric Function/1  "<beta>"
  Bus Selector/3 -> Trigonometric Function1/1  "<alpha>"
  Bus Selector/1 -> Product/1  "<V>"
  Trigonometric Function/1 -> Product/2
  Trigonometric Function1/1 -> Product/3
  Bus Selector1/2 -> Trigonometric Function2/1  "<beta>"
  Bus Selector1/1 -> Product1/1  "<V>"
  Trigonometric Function2/1 -> Product1/2
  Bus Selector2/2 -> Trigonometric Function3/1  "<beta>"
  Bus Selector2/3 -> Trigonometric Function4/1  "<alpha>"
  Bus Selector2/1 -> Product2/1  "<V>"
  Trigonometric Function3/1 -> Product2/2
  Trigonometric Function4/1 -> Product2/3
  Product/1 -> Mux/1
  Product1/1 -> Mux/2
  Product2/1 -> Mux/3
  In1/1 -> Selector1/1
  Mux/1 -> Out1/1

== system Han_HQ_Sim_FB/AircraftModel/Make_Data/Subsystem2/get_psi ==
  x : Inport
  Demux7 : Demux  Outputs=6
  Integrator : Integrator  InitialCondition=90*pi/180
  Product : Product  Inputs=**/  RndMeth=Zero
  Product1 : Product  Inputs=**/  RndMeth=Zero
  Selector4 : Selector  InputPortWidth=8  IndexOptions=Index vector (dialog)  Indices=[3 8 4 7 8 4]  OutputSizes=1
  Sum : Sum  Inputs=|++
  Trigonometric Function : Trigonometry
  Trigonometric Function1 : Trigonometry  Operator=cos
  Trigonometric Function2 : Trigonometry  Operator=cos
  Trigonometric Function3 : Trigonometry  Operator=cos
  psi : Outport
  wires:
  Integrator/1 -> psi/1  "psi"
  x/1 -> Selector4/1
  Sum/1 -> Integrator/1  "psi_dt"
  Product1/1 -> Sum/2
  Demux7/5 -> Trigonometric Function2/1
  Trigonometric Function3/1 -> Product1/3
  Trigonometric Function2/1 -> Product1/2
  Demux7/4 -> Product1/1
  Demux7/6 -> Trigonometric Function3/1
  Product/1 -> Sum/1
  Trigonometric Function1/1 -> Product/3
  Trigonometric Function/1 -> Product/2
  Demux7/1 -> Product/1
  Demux7/3 -> Trigonometric Function1/1
  Demux7/2 -> Trigonometric Function/1
  Selector4/1 -> Demux7/1

== system Han_HQ_Sim_FB/Scopes/Directional_Task_Data/Task6/LogicA ==
  In1 : Inport
  Compare To Constant : simulink/Logic and Bit Operations/Compare To Constant  relop=<=  const=2.5  OutDataTypeStr=uint8  ZeroCross=off
  Compare To Constant1 : simulink/Logic and Bit Operations/Compare To Constant  relop=>=  const=1.5  OutDataTypeStr=uint8  ZeroCross=off
  Data Type Conversion : DataTypeConversion
  Logical Operator : Logic  AllPortsSameDT=off  OutDataTypeStr=boolean
  Out1 : Outport
  wires:
  Data Type Conversion/1 -> Out1/1
  In1/1 -> Compare To Constant1/1, Compare To Constant/1
  Logical Operator/1 -> Data Type Conversion/1
  Compare To Constant1/1 -> Logical Operator/2
  Compare To Constant/1 -> Logical Operator/1

== system Han_HQ_Sim_FB/Scopes/Directional_Task_Data/Task6/LogicD ==
  In1 : Inport
  Compare To Constant : simulink/Logic and Bit Operations/Compare To Constant  relop=<=  const=2.25  OutDataTypeStr=uint8  ZeroCross=off
  Compare To Constant1 : simulink/Logic and Bit Operations/Compare To Constant  relop=>=  const=1.75  OutDataTypeStr=uint8  ZeroCross=off
  Data Type Conversion2 : DataTypeConversion
  Logical Operator2 : Logic  AllPortsSameDT=off  OutDataTypeStr=boolean
  Out1 : Outport
  wires:
  Data Type Conversion2/1 -> Out1/1
  In1/1 -> Compare To Constant/1, Compare To Constant1/1
  Logical Operator2/1 -> Data Type Conversion2/1
  Compare To Constant1/1 -> Logical Operator2/2
  Compare To Constant/1 -> Logical Operator2/1

== system Han_HQ_Sim_FB/Scopes/Directional_Task_Data/Task7/LogicA ==
  In2 : Inport
  In3 : Inport  Port=2
  Compare To Constant : simulink/Logic and Bit Operations/Compare To Constant  relop=<=  const=.5  OutDataTypeStr=uint8  ZeroCross=off
  Compare To Constant1 : simulink/Logic and Bit Operations/Compare To Constant  relop=>=  const=-0.5  OutDataTypeStr=uint8  ZeroCross=off
  Data Type Conversion : DataTypeConversion
  Logical Operator : Logic  Inputs=3  AllPortsSameDT=off  OutDataTypeStr=boolean
  Out1 : Outport
  wires:
  Data Type Conversion/1 -> Out1/1
  In3/1 -> Logical Operator/3
  In2/1 -> Compare To Constant/1, Compare To Constant1/1
  Compare To Constant/1 -> Logical Operator/1
  Compare To Constant1/1 -> Logical Operator/2
  Logical Operator/1 -> Data Type Conversion/1

== system Han_HQ_Sim_FB/Scopes/Directional_Task_Data/Task7/LogicD ==
  In1 : Inport
  In2 : Inport  Port=2
  Compare To Constant3 : simulink/Logic and Bit Operations/Compare To Constant  relop=<=  const=0.25  OutDataTypeStr=uint8  ZeroCross=off
  Compare To Constant4 : simulink/Logic and Bit Operations/Compare To Constant  relop=>=  const=-0.25  OutDataTypeStr=uint8  ZeroCross=off
  Data Type Conversion3 : DataTypeConversion
  Logical Operator2 : Logic  Inputs=3  AllPortsSameDT=off  OutDataTypeStr=boolean
  Out1 : Outport
  wires:
  Data Type Conversion3/1 -> Out1/1
  In2/1 -> Compare To Constant3/1, Compare To Constant4/1
  In1/1 -> Logical Operator2/1
  Compare To Constant4/1 -> Logical Operator2/3
  Compare To Constant3/1 -> Logical Operator2/2
  Logical Operator2/1 -> Data Type Conversion3/1

== system Han_HQ_Sim_FB/Scopes/Lateral_Task_Data/Task3/LogicA ==
  In1 : Inport
  Compare To Constant : simulink/Logic and Bit Operations/Compare To Constant  relop=<=  const=11  OutDataTypeStr=uint8  ZeroCross=off
  Compare To Constant1 : simulink/Logic and Bit Operations/Compare To Constant  relop=>=  const=9  OutDataTypeStr=uint8  ZeroCross=off
  Data Type Conversion : DataTypeConversion
  Logical Operator : Logic  AllPortsSameDT=off  OutDataTypeStr=boolean
  Out1 : Outport
  wires:
  Compare To Constant/1 -> Logical Operator/1
  Compare To Constant1/1 -> Logical Operator/2
  Logical Operator/1 -> Data Type Conversion/1
  In1/1 -> Compare To Constant/1, Compare To Constant1/1
  Data Type Conversion/1 -> Out1/1

== system Han_HQ_Sim_FB/Scopes/Lateral_Task_Data/Task3/LogicD ==
  In1 : Inport
  Compare To Constant : simulink/Logic and Bit Operations/Compare To Constant  relop=<=  const=10.5  OutDataTypeStr=uint8  ZeroCross=off
  Compare To Constant1 : simulink/Logic and Bit Operations/Compare To Constant  relop=>=  const=9.5  OutDataTypeStr=uint8  ZeroCross=off
  Data Type Conversion2 : DataTypeConversion
  Logical Operator2 : Logic  AllPortsSameDT=off  OutDataTypeStr=boolean
  Out1 : Outport
  wires:
  Compare To Constant/1 -> Logical Operator2/1
  Compare To Constant1/1 -> Logical Operator2/2
  Logical Operator2/1 -> Data Type Conversion2/1
  In1/1 -> Compare To Constant1/1, Compare To Constant/1
  Data Type Conversion2/1 -> Out1/1

== system Han_HQ_Sim_FB/Scopes/Lateral_Task_Data/Task4/LogicA ==
  In2 : Inport
  In3 : Inport  Port=2
  Compare To Constant : simulink/Logic and Bit Operations/Compare To Constant  relop=<=  const=-9  OutDataTypeStr=uint8  ZeroCross=off
  Compare To Constant1 : simulink/Logic and Bit Operations/Compare To Constant  relop=>=  const=-11  OutDataTypeStr=uint8  ZeroCross=off
  Data Type Conversion : DataTypeConversion
  Logical Operator : Logic  Inputs=3  AllPortsSameDT=off  OutDataTypeStr=boolean
  Out1 : Outport
  wires:
  Logical Operator/1 -> Data Type Conversion/1
  Compare To Constant1/1 -> Logical Operator/2
  Compare To Constant/1 -> Logical Operator/1
  In2/1 -> Compare To Constant1/1, Compare To Constant/1
  In3/1 -> Logical Operator/3
  Data Type Conversion/1 -> Out1/1

== system Han_HQ_Sim_FB/Scopes/Lateral_Task_Data/Task4/LogicD ==
  In1 : Inport
  In2 : Inport  Port=2
  Compare To Constant3 : simulink/Logic and Bit Operations/Compare To Constant  relop=<=  const=-9.5  OutDataTypeStr=uint8  ZeroCross=off
  Compare To Constant4 : simulink/Logic and Bit Operations/Compare To Constant  relop=>=  const=-10.5  OutDataTypeStr=uint8  ZeroCross=off
  Data Type Conversion3 : DataTypeConversion
  Logical Operator2 : Logic  Inputs=3  AllPortsSameDT=off  OutDataTypeStr=boolean
  Out1 : Outport
  wires:
  Logical Operator2/1 -> Data Type Conversion3/1
  Compare To Constant3/1 -> Logical Operator2/2
  Compare To Constant4/1 -> Logical Operator2/3
  In1/1 -> Logical Operator2/1
  In2/1 -> Compare To Constant4/1, Compare To Constant3/1
  Data Type Conversion3/1 -> Out1/1

== system Han_HQ_Sim_FB/Scopes/Lateral_Task_Data/Task5/LogicA ==
  In2 : Inport
  In3 : Inport  Port=2
  Compare To Constant : simulink/Logic and Bit Operations/Compare To Constant  relop=<=  const=1  OutDataTypeStr=uint8  ZeroCross=off
  Compare To Constant1 : simulink/Logic and Bit Operations/Compare To Constant  relop=>=  const=-1  OutDataTypeStr=uint8  ZeroCross=off
  Data Type Conversion : DataTypeConversion
  Logical Operator : Logic  Inputs=3  AllPortsSameDT=off  OutDataTypeStr=boolean
  Out1 : Outport
  wires:
  Logical Operator/1 -> Data Type Conversion/1
  Compare To Constant1/1 -> Logical Operator/2
  Compare To Constant/1 -> Logical Operator/1
  In2/1 -> Compare To Constant1/1, Compare To Constant/1
  In3/1 -> Logical Operator/3
  Data Type Conversion/1 -> Out1/1

== system Han_HQ_Sim_FB/Scopes/Lateral_Task_Data/Task5/LogicD ==
  In1 : Inport
  In2 : Inport  Port=2
  Compare To Constant3 : simulink/Logic and Bit Operations/Compare To Constant  relop=<=  const=0.5  OutDataTypeStr=uint8  ZeroCross=off
  Compare To Constant4 : simulink/Logic and Bit Operations/Compare To Constant  relop=>=  const=-0.5  OutDataTypeStr=uint8  ZeroCross=off
  Data Type Conversion3 : DataTypeConversion
  Logical Operator2 : Logic  Inputs=3  AllPortsSameDT=off  OutDataTypeStr=boolean
  Out1 : Outport
  wires:
  Logical Operator2/1 -> Data Type Conversion3/1
  Compare To Constant3/1 -> Logical Operator2/2
  Compare To Constant4/1 -> Logical Operator2/3
  In1/1 -> Logical Operator2/1
  In2/1 -> Compare To Constant4/1, Compare To Constant3/1
  Data Type Conversion3/1 -> Out1/1

== system Han_HQ_Sim_FB/Scopes/Longitudinal_Task_Data/Task1/LogicA ==
  In1 : Inport
  Compare To Constant : simulink/Logic and Bit Operations/Compare To Constant  relop=<=  const=6+(tht*180/pi)  OutDataTypeStr=uint8  ZeroCross=off
  Compare To Constant1 : simulink/Logic and Bit Operations/Compare To Constant  relop=>=  const=4+(tht*180/pi)  OutDataTypeStr=uint8  ZeroCross=off
  Data Type Conversion : DataTypeConversion
  Logical Operator : Logic  AllPortsSameDT=off  OutDataTypeStr=boolean
  Out1 : Outport
  wires:
  Compare To Constant/1 -> Logical Operator/1
  Compare To Constant1/1 -> Logical Operator/2
  Logical Operator/1 -> Data Type Conversion/1
  In1/1 -> Compare To Constant/1, Compare To Constant1/1
  Data Type Conversion/1 -> Out1/1

== system Han_HQ_Sim_FB/Scopes/Longitudinal_Task_Data/Task1/LogicD ==
  In1 : Inport
  Compare To Constant : simulink/Logic and Bit Operations/Compare To Constant  relop=<=  const=5.5+(tht*180/pi)  OutDataTypeStr=uint8  ZeroCross=off
  Compare To Constant1 : simulink/Logic and Bit Operations/Compare To Constant  relop=>=  const=4.5+(tht*180/pi)  OutDataTypeStr=uint8  ZeroCross=off
  Data Type Conversion2 : DataTypeConversion
  Logical Operator2 : Logic  AllPortsSameDT=off  OutDataTypeStr=boolean
  Out1 : Outport
  wires:
  Compare To Constant/1 -> Logical Operator2/1
  Compare To Constant1/1 -> Logical Operator2/2
  Logical Operator2/1 -> Data Type Conversion2/1
  In1/1 -> Compare To Constant1/1, Compare To Constant/1
  Data Type Conversion2/1 -> Out1/1

== system Han_HQ_Sim_FB/Scopes/Longitudinal_Task_Data/Task2/LogicA ==
  In1 : Inport
  In2 : Inport  Port=2
  Compare To Constant2 : simulink/Logic and Bit Operations/Compare To Constant  relop=<=  const=1+(tht*180/pi)  OutDataTypeStr=uint8  ZeroCross=off
  Compare To Constant3 : simulink/Logic and Bit Operations/Compare To Constant  relop=>=  const=-1+(tht*180/pi)  OutDataTypeStr=uint8  ZeroCross=off
  Data Type Conversion : DataTypeConversion
  Logical Operator : Logic  Inputs=3  AllPortsSameDT=off  OutDataTypeStr=boolean
  Out1 : Outport
  wires:
  Logical Operator/1 -> Data Type Conversion/1
  Compare To Constant3/1 -> Logical Operator/2
  Compare To Constant2/1 -> Logical Operator/1
  In1/1 -> Compare To Constant2/1, Compare To Constant3/1
  In2/1 -> Logical Operator/3
  Data Type Conversion/1 -> Out1/1

== system Han_HQ_Sim_FB/Scopes/Longitudinal_Task_Data/Task2/LogicD ==
  In1 : Inport
  In2 : Inport  Port=2
  Compare To Constant : simulink/Logic and Bit Operations/Compare To Constant  relop=<=  const=0.5+(tht*180/pi)  OutDataTypeStr=uint8  ZeroCross=off
  Compare To Constant1 : simulink/Logic and Bit Operations/Compare To Constant  relop=>=  const=-0.5+(tht*180/pi)  OutDataTypeStr=uint8  ZeroCross=off
  Data Type Conversion3 : DataTypeConversion
  Logical Operator2 : Logic  Inputs=3  AllPortsSameDT=off  OutDataTypeStr=boolean
  Out1 : Outport
  wires:
  Logical Operator2/1 -> Data Type Conversion3/1
  Compare To Constant/1 -> Logical Operator2/2
  Compare To Constant1/1 -> Logical Operator2/3
  In1/1 -> Logical Operator2/1
  In2/1 -> Compare To Constant/1, Compare To Constant1/1
  Data Type Conversion3/1 -> Out1/1

== system Han_HQ_Sim_FB/AircraftModel/Make_Data/Earth Axis/Subsystem1/Euler Rates ==
  p q r : Inport
  phi theta psi1 : Inport  Port=2
  Mux1 : Mux  Inputs=[3 3 3]
  Mux2 : Mux  Inputs=3
  phidot : Fcn  Expr=u[1]+(u[2]*u[4]+u[3]*u[7])*(u[5]/u[8])
  psidot : Fcn  Expr=(u[2]*u[4]+u[3]*u[7])/u[8]
  sincos : Trigonometry  Operator=sincos
  thetadot : Fcn  Expr=u[2]*u[7]-u[3]*u[4]
  phidot thetadot psi : Outport  InitialOutput=0
  wires:
  Mux1/1 -> psidot/1, phidot/1, thetadot/1
  p q r/1 -> Mux1/1
  phi theta psi1/1 -> sincos/1
  psidot/1 -> Mux2/3
  thetadot/1 -> Mux2/2
  phidot/1 -> Mux2/1
  Mux2/1 -> phidot thetadot psi/1
  sincos/1 -> Mux1/2
  sincos/2 -> Mux1/3

== system Han_HQ_Sim_FB/AircraftModel/Make_Data/Earth Axis/Subsystem1/Make DCM ==
  In1 : Inport  PortDimensions=3
  Fcn11 : Fcn  Expr=u(5)*u(4)
  Fcn12 : Fcn  Expr=u(5)*u(1)
  Fcn13 : Fcn  Expr=-u(2)
  Fcn21 : Fcn  Expr=u(3)*u(2)*u(4) - u(6)*u(1)
  Fcn22 : Fcn  Expr=u(3)*u(2)*u(1) + u(6)*u(4)
  Fcn23 : Fcn  Expr=u(3)*u(5)
  Fcn31 : Fcn  Expr=u(6)*u(2)*u(4) + u(3)*u(1)
  Fcn32 : Fcn  Expr=u(6)*u(2)*u(1) - u(3)*u(4)
  Fcn33 : Fcn  Expr=u(6)*u(5)
  Make 3x3 : Subsystem
  Mux : Mux  Inputs=2
  sincos : Trigonometry  Operator=sincos
  Out1 : Outport  PortDimensions=[3,3]
  wires:
  In1/1 -> sincos/1
  Make 3x3/1(Matrix) -> Out1/1
  sincos/1 -> Mux/1
  sincos/2 -> Mux/2
  Mux/1 -> Fcn32/1, Fcn33/1, Fcn31/1, Fcn23/1, Fcn22/1, Fcn11/1, Fcn12/1, Fcn13/1, Fcn21/1
  Fcn11/1 -> Make 3x3/1(M11)
  Fcn12/1 -> Make 3x3/2(M12)
  Fcn13/1 -> Make 3x3/3(M13)
  Fcn21/1 -> Make 3x3/4(M21)
  Fcn22/1 -> Make 3x3/5(M22)
  Fcn23/1 -> Make 3x3/6(M23)
  Fcn31/1 -> Make 3x3/7(M31)
  Fcn32/1 -> Make 3x3/8(M32)
  Fcn33/1 -> Make 3x3/9(M33)

== system Han_HQ_Sim_FB/AircraftModel/Make_Data/Earth Axis/Subsystem1/Make DCM/Make 3x3 ==
  M11 : Inport  PortDimensions=1
  M12 : Inport  Port=2  PortDimensions=1
  M13 : Inport  Port=3  PortDimensions=1
  M21 : Inport  Port=4  PortDimensions=1
  M22 : Inport  Port=5  PortDimensions=1
  M23 : Inport  Port=6  PortDimensions=1
  M31 : Inport  Port=7  PortDimensions=1
  M32 : Inport  Port=8  PortDimensions=1
  M33 : Inport  Port=9  PortDimensions=1
  Reshape (9) to [3x3] column-major : Reshape  OutputDimensionality=Customize  OutputDimensions=[3,3]
  Vector Concatenate : Concatenate  NumInputs=9
  Matrix : Outport  PortDimensions=[3 3]
  wires:
  M33/1 -> Vector Concatenate/9
  M23/1 -> Vector Concatenate/8
  M13/1 -> Vector Concatenate/7
  M32/1 -> Vector Concatenate/6
  Reshape (9) to [3x3] column-major/1 -> Matrix/1
  M22/1 -> Vector Concatenate/5
  M12/1 -> Vector Concatenate/4
  M31/1 -> Vector Concatenate/3
  M21/1 -> Vector Concatenate/2
  M11/1 -> Vector Concatenate/1
  Vector Concatenate/1 -> Reshape (9) to [3x3] column-major/1
